simulink model "horno_alta_temperatura"  (R2015a)
settings: Solver=ode45  StartTime=0.0  StopTime=2000  RelTol=1e-3
libraries: simulink x2
settings Model: Creator=m4v  LastModifiedBy=m4v

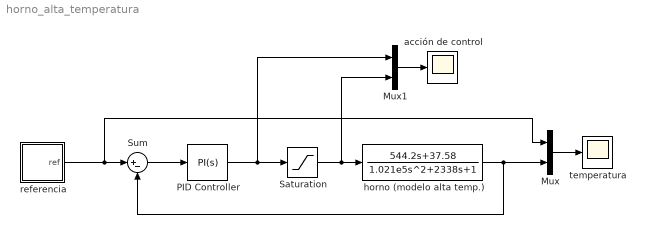
== system horno_alta_temperatura ==
  Mux : Mux  Inputs=2
  Mux1 : Mux  Inputs=2
  PID Controller : simulink/Continuous/PID Controller  Controller=PI  TimeDomain=Continuous-time  SampleTime=-1  IntegratorMethod=Forward Euler  FilterMethod=Forward Euler  Form=Parallel  UseFilter=on  ControllerParametersSource=internal  P=3.5  I=0.0012  D=0  N=100  InitialConditionSource=internal  InitialConditionForIntegrator=0  InitialConditionForFilter=0  ExternalReset=none  LimitOutput=off  UpperSaturationLimit=100  LowerSaturationLimit=0  LinearizeAsGain=on  AntiWindupMode=clamping  Kb=1  TrackingMode=off  Kt=1  PParamMin=[]  PParamMax=[]  IParamMin=[]  IParamMax=[]  DParamMin=[]  DParamMax=[]  NParamMin=[]  NParamMax=[]  KbParamMin=[]  KbParamMax=[]  KtParamMin=[]  KtParamMax=[]  POutMin=[]  POutMax=[]  IOutMin=[]  IOutMax=[]  DOutMin=[]  DOutMax=[]  NOutMin=[]  NOutMax=[]  KbOutMin=[]  KbOutMax=[]  KtOutMin=[]  KtOutMax=[]  IntegratorOutMin=[]  IntegratorOutMax=[]  FilterOutMin=[]  FilterOutMax=[]  SumOutMin=[]  SumOutMax=[]  SumI1OutMin=[]  SumI1OutMax=[]  SumI2OutMin=[]  SumI2OutMax=[]  SumI3OutMin=[]  SumI3OutMax=[]  SumDOutMin=[]  SumDOutMax=[]  SaturationOutMin=[]  SaturationOutMax=[]  IntegratorContinuousStateAttributes=''  IntegratorStateMustResolveToSignalObject=off  IntegratorRTWStateStorageClass=Auto  FilterContinuousStateAttributes=''  FilterStateMustResolveToSignalObject=off  FilterRTWStateStorageClass=Auto  DifferentiatorICPrevScaledInput=0  DifferentiatorOutMin=[]  DifferentiatorOutMax=[]
  Saturation : Saturate  UpperLimit=100  LowerLimit=0  ZeroCross=off
  Sum : Sum  Inputs=|+-
  acción de control : Scope
      settings: TimeRange=8000  YMin=0  YMax=80
  horno (modelo alta temp.) : TransferFcn  Numerator=[544.2 37.58]  Denominator=[1.021e5 2338 1]
  referencia : Subsystem
  temperatura : Scope
      settings: TimeRange=2000  YMin=0  YMax=900  SampleInput=on  SampleTime=1
  wires:
  Sum/1 -> PID Controller/1
  Mux1/1 -> acción de control/1
  PID Controller/1 -> Mux1/1, Saturation/1
  Saturation/1 -> Mux1/2, horno (modelo alta temp.)/1
  horno (modelo alta temp.)/1 -> Sum/2, Mux/2
  Mux/1 -> temperatura/1
  referencia/1(ref) -> Mux/1, Sum/1

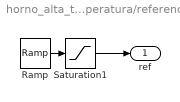
== system horno_alta_temperatura/referencia ==
  Ramp : simulink/Sources/Ramp  slope=0.8  start=0  X0=0
  Saturation1 : Saturate  UpperLimit=800  LowerLimit=0
  ref : Outport
  wires:
  Ramp/1 -> Saturation1/1
  Saturation1/1 -> ref/1
